simulink model "Model_copied"  (R2015a)
settings: Solver=ode45  StartTime=0.0  StopTime=10.0  RelTol=1e-3
values from neighbouring files (symbols this model uses):
  Ch = 9    [ss_model.m]    (also in synthesis.m)
  Cm = 6    [ss_model.m]    (also in synthesis.m)
  Ke = -1.0000e+05    (= -100000)    [ss_model.m]    (also in synthesis.m)
  Kh = 625    [ss_model.m]    (also in synthesis.m)
  Km = 281    [ss_model.m]    (also in synthesis.m)
  L = 0.0220    (= 0.022)    [ss_model.m]    (also in synthesis.m)
  M1 = 1.35    [synthesis.m]
  M2 = 1.35    [synthesis.m]
  R = 1.3    [ss_model.m]    (also in synthesis.m)
settings Model: CovModelRefEnable=off  Creator=gsavaia  LastModifiedBy=user
settings DataIOCC: SaveFormat=Dataset
settings HardwareCC: ProdBitPerPointer=64  ProdLargestAtomicFloat=Float  ProdIntDivRoundTo=Zero  ProdEndianess=LittleEndian  ProdHWDeviceType=Specified
settings GRTTargetCC: GeneratePreprocessorConditionals=Use local settings

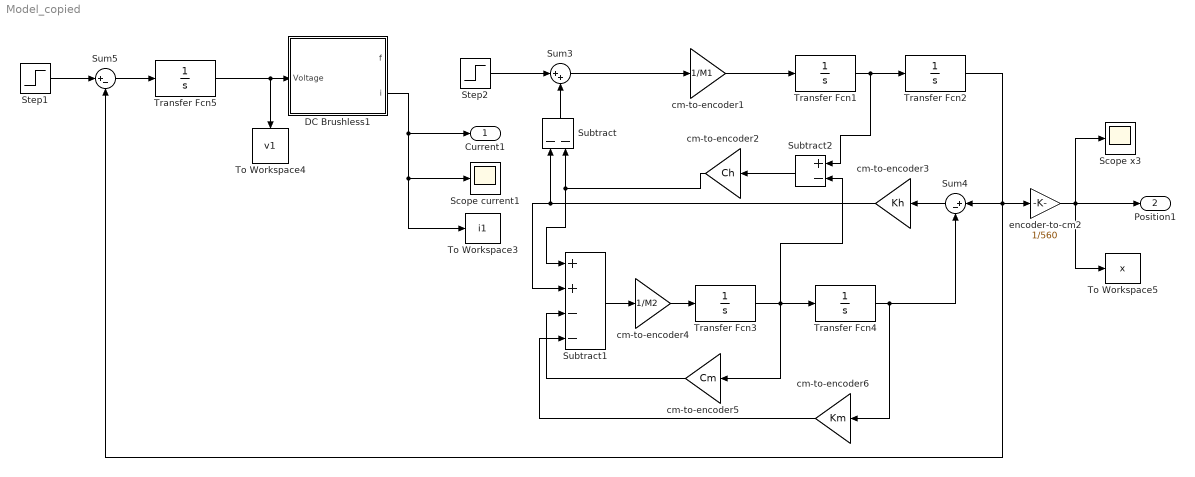
== system Model_copied ==
  DC Brushless1 : Subsystem
  Scope x3 : Scope
      settings: YMin=-0.25393  YMax=2.28535  SaveName=ScopeData5
  Scope current1 : Scope
      settings: YMin=-0.525  YMax=4.725  SaveName=ScopeData3
  Step1 : Step  SampleTime=0
  Step2 : Step  SampleTime=0
  Subtract : Sum  Inputs=--
  Subtract1 : Sum  Inputs=++--
  Subtract2 : Sum  Inputs=+-
  Sum3 : Sum  Inputs=|++
  Sum4 : Sum  Inputs=|+-
  Sum5 : Sum  Inputs=|+-
  To Workspace3 : ToWorkspace  VariableName=i1  SaveFormat=Timeseries  SampleTime=-1
  To Workspace4 : ToWorkspace  VariableName=v1  SaveFormat=Timeseries  SampleTime=-1
  To Workspace5 : ToWorkspace  VariableName=x  SaveFormat=Timeseries  SampleTime=-1
  Transfer Fcn{1..5} (5 alike) : TransferFcn  Numerator=1  Denominator=[1 0]
  cm-to-encoder1 : Gain  Gain=1/M1
  cm-to-encoder2 : Gain  Gain=Ch
  cm-to-encoder3 : Gain  Gain=Kh
  cm-to-encoder4 : Gain  Gain=1/M2
  cm-to-encoder5 : Gain  Gain=Cm
  cm-to-encoder6 : Gain  Gain=Km
  encoder-to-cm2 : Gain  Gain=1/560
  Current1 : Outport
  Position1 : Outport  Port=2
  wires:
  cm-to-encoder3/1 -> Subtract1/2, Subtract/1
  cm-to-encoder1/1 -> Transfer Fcn1/1
  Subtract/1 -> Sum3/2
  Transfer Fcn1/1 -> Subtract2/1, Transfer Fcn2/1
  Transfer Fcn2/1 -> encoder-to-cm2/1, Sum5/2, Sum4/1
  Subtract2/1 -> cm-to-encoder2/1
  cm-to-encoder2/1 -> Subtract/2, Subtract1/1
  Sum4/1 -> cm-to-encoder3/1
  Subtract1/1 -> cm-to-encoder4/1
  cm-to-encoder4/1 -> Transfer Fcn3/1
  Transfer Fcn3/1 -> Subtract2/2, cm-to-encoder5/1, Transfer Fcn4/1
  cm-to-encoder5/1 -> Subtract1/3
  Transfer Fcn4/1 -> Sum4/2, cm-to-encoder6/1
  cm-to-encoder6/1 -> Subtract1/4
  Sum3/1 -> cm-to-encoder1/1
  DC Brushless1/2(i) -> Current1/1, To Workspace3/1, Scope current1/1
  Transfer Fcn5/1 -> To Workspace4/1, DC Brushless1/1("Voltage ")
  Step1/1 -> Sum5/1
  Sum5/1 -> Transfer Fcn5/1
  encoder-to-cm2/1 -> Position1/1, To Workspace5/1, Scope x3/1
  Step2/1 -> Sum3/1

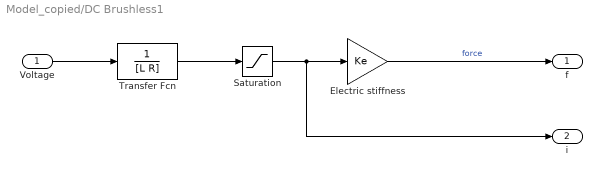
== system Model_copied/DC Brushless1 ==
  "Voltage " : Inport
  Electric stiffness : Gain  Gain=Ke
  Saturation : Saturate  UpperLimit=4.2  LowerLimit=-10
  Transfer Fcn : TransferFcn  Denominator=[L R]
  "f " : Outport
  i : Outport  Port=2
  wires:
  "Voltage "/1 -> Transfer Fcn/1
  Electric stiffness/1 -> "f "/1  "force"
  Transfer Fcn/1 -> Saturation/1
  Saturation/1 -> i/1, Electric stiffness/1
